simulink subsystem "TEORIA_Non_linear_continuous_drone_plant"  (R2020a)
settings: Solver=VariableStepAuto  StartTime=0.0  StopTime=10.0  RelTol=1e-3
settings Model: Creator=augus  LastModifiedBy=augus

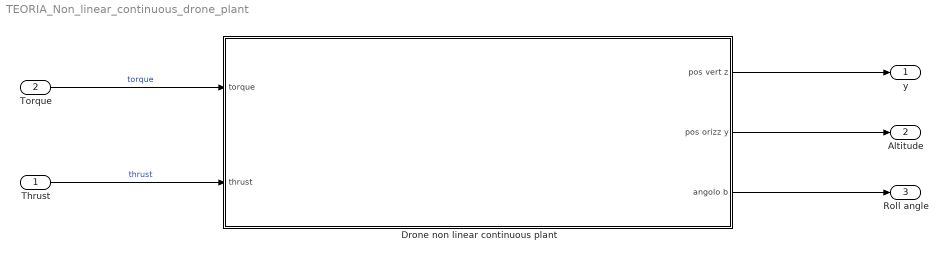
== system TEORIA_Non_linear_continuous_drone_plant ==
  Thrust : Inport  Tag=torque  Description=torque
  Torque : Inport  Tag=thrust  Description=thrust  Port=2
  Drone non linear continuous plant : Subsystem
  y : Outport  Tag=y position  Description=y position
  Altitude : Outport  Tag=z position  Description=z position  Port=2
  Roll angle : Outport  Tag=roll angle  Description=roll angle  Port=3
  wires:
  Torque/1 -> Drone non linear continuous plant/1(torque)  "torque"
  Thrust/1 -> Drone non linear continuous plant/2(thrust)  "thrust"
  Drone non linear continuous plant/3(angolo b) -> Roll angle/1
  Drone non linear continuous plant/2(pos orizz y) -> Altitude/1
  Drone non linear continuous plant/1(pos vert z) -> y/1

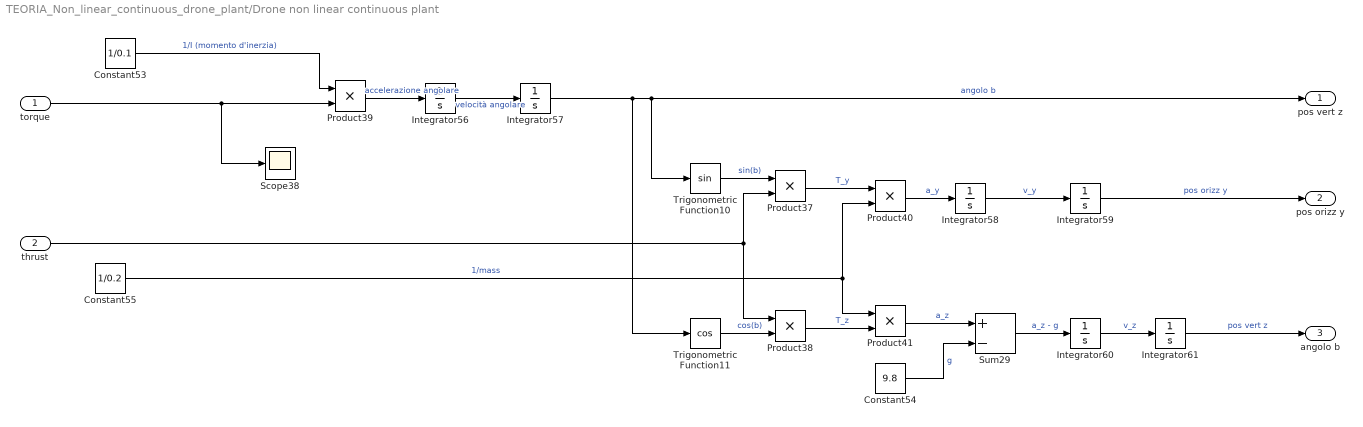
== system TEORIA_Non_linear_continuous_drone_plant/Drone non linear continuous plant ==
  torque : Inport
  thrust : Inport  Port=2
  Constant53 : Constant  Value=1/0.1
  Constant54 : Constant  Value=9.8
  Constant55 : Constant  Value=1/0.2
  Integrator{56..61} (6 alike) : Integrator
  Product{37..41} (5 alike) : Product
  Scope38 : Scope
  Sum29 : Sum  Inputs=+-
  Trigonometric Function10 : Trigonometry
  Trigonometric Function11 : Trigonometry  Operator=cos
  pos vert z : Outport
  pos orizz y : Outport  Port=2
  angolo b : Outport  Port=3
  wires:
  Integrator60/1 -> Integrator61/1  "v_z"
  Integrator57/1 -> pos vert z/1, Trigonometric Function10/1, Trigonometric Function11/1  "angolo b"
  Constant55/1 -> Product41/1, Product40/2  "1/mass"
  torque/1 -> Product39/2, Scope38/1
  Product38/1 -> Product41/2  "T_z"
  thrust/1 -> Product38/1, Product37/2
  Constant53/1 -> Product39/1  "1/I (momento d'inerzia)"
  Product39/1 -> Integrator56/1  "accelerazione angolare"
  Integrator56/1 -> Integrator57/1  "velocità angolare"
  Product37/1 -> Product40/1  "T_y"
  Trigonometric Function11/1 -> Product38/2  "cos(b)"
  Product41/1 -> Sum29/1  "a_z"
  Integrator58/1 -> Integrator59/1  "v_y"
  Trigonometric Function10/1 -> Product37/1  "sin(b)"
  Sum29/1 -> Integrator60/1  "a_z - g"
  Product40/1 -> Integrator58/1  "a_y"
  Constant54/1 -> Sum29/2  "g"
  Integrator59/1 -> pos orizz y/1  "pos orizz y"
  Integrator61/1 -> angolo b/1  "pos vert z"
